simulink library "Chassis_Alpha_org"  (Simulink 10.0)
settings: Solver=ode45  StartTime=0.0  StopTime=10.0  RelTol=1e-3  EnableMultiTasking=on
undefined symbols (not defined in the file): Chassis, lat0, latMean, lon0, Suspension, transMatrix, v_ds, xx_ds, yy_ds, z_accel, z_dist, z_elevTube, z_height
libraries: simulink x4, Chassis_Alpha x2
Description:
  | Copyright 2013-2014 The MathWorks, Inc.
settings Model: Creator=mbrauer  LastModifiedBy=annonymous

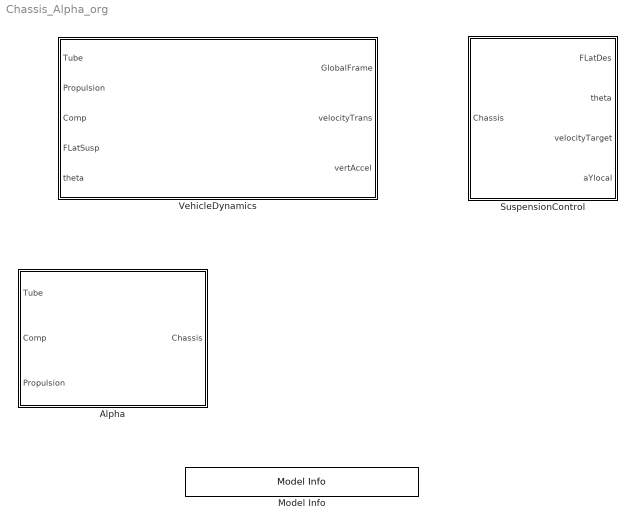
== system Chassis_Alpha_org ==
  Alpha : Subsystem
  Model Info : simulink/Model-Wide Utilities/Model Info  Frame=on  DisplayStringWithTags=%<Description>  HorizontalTextAlignment=Center  LeftAlignmentValue=0.5
  SuspensionControl : Subsystem
  VehicleDynamics : Subsystem

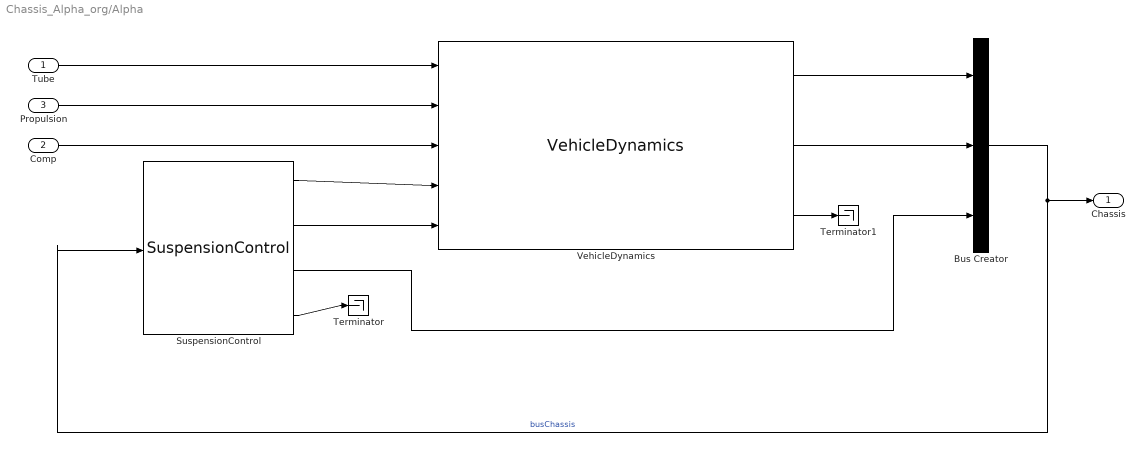
== system Chassis_Alpha_org/Alpha ==
  "Tube " : Inport
  Comp : Inport  Port=2
  Propulsion : Inport  Port=3
  Bus Creator : BusCreator  Inputs=3  NonVirtualBus=on
  SuspensionControl : Chassis_Alpha/SuspensionControl  SystemSampleTime=-1  Latency=0  AutoFrameSizeCalculation=off
  Terminator : Terminator
  Terminator1 : Terminator
  VehicleDynamics : Chassis_Alpha/VehicleDynamics  SystemSampleTime=-1  Latency=0  AutoFrameSizeCalculation=off
  Chassis : Outport
  wires:
  SuspensionControl/4 -> Terminator/1
  Bus Creator/1 -> SuspensionControl/1, Chassis/1  "busChassis"
  Comp/1 -> VehicleDynamics/3
  "Tube "/1 -> VehicleDynamics/1
  VehicleDynamics/1 -> Bus Creator/1
  VehicleDynamics/2 -> Bus Creator/2
  Propulsion/1 -> VehicleDynamics/2
  SuspensionControl/1 -> VehicleDynamics/4
  SuspensionControl/2 -> VehicleDynamics/5
  SuspensionControl/3 -> Bus Creator/3
  VehicleDynamics/3 -> Terminator1/1

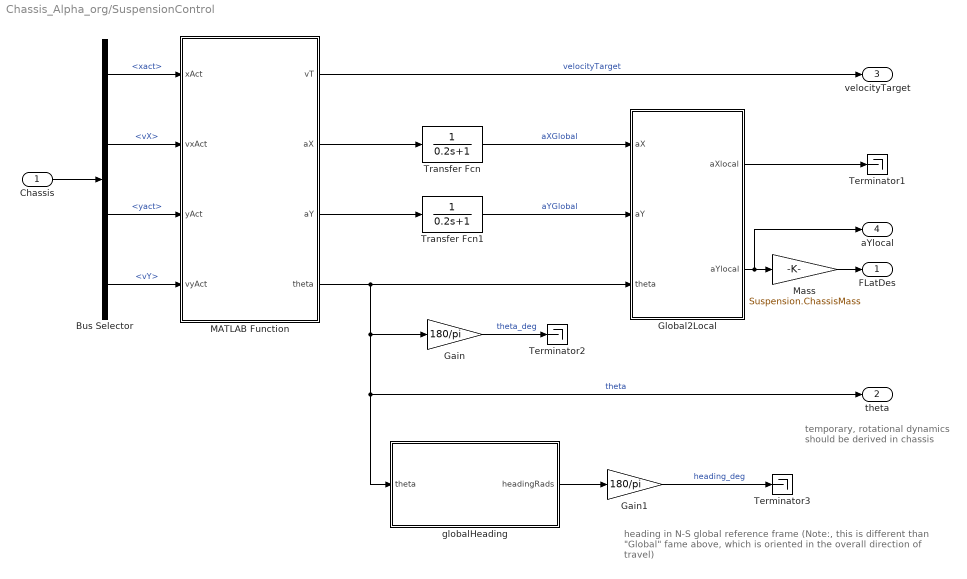
== system Chassis_Alpha_org/SuspensionControl ==
  note: temporary, rotational dynamics
      | should be derived in chassis
  note: heading in N-S global reference frame
      | (Note:, this is different than "Global" fame above, which is oriented
      | in the overall direction of travel)
  Chassis : Inport
  Bus Selector : BusSelector  OutputSignals=GlobalFrame.xact,GlobalFrame.vX,GlobalFrame.yact,GlobalFrame.vY
  Gain : Gain  Gain=180/pi
  Gain1 : Gain  Gain=180/pi
  Global2Local : MATLAB Function  TreatAsAtomicUnit=on
  MATLAB Function : MATLAB Function  TreatAsAtomicUnit=on
  Mass : Gain  Gain=Suspension.ChassisMass
  Terminator1 : Terminator
  Terminator2 : Terminator
  Terminator3 : Terminator
  Transfer Fcn : TransferFcn  Denominator=[0.2 1]
  Transfer Fcn1 : TransferFcn  Denominator=[0.2 1]
  globalHeading : MATLAB Function  TreatAsAtomicUnit=on
  FLatDes : Outport
  theta : Outport  Port=2
  velocityTarget : Outport  Port=3
  aYlocal : Outport  Port=4
  wires:
  Gain1/1 -> Terminator3/1  "heading_deg"
  globalHeading/1(headingRads) -> Gain1/1
  MATLAB Function/2(aX) -> Transfer Fcn/1
  MATLAB Function/3(aY) -> Transfer Fcn1/1
  Transfer Fcn/1 -> Global2Local/1(aX)  "aXGlobal"
  Transfer Fcn1/1 -> Global2Local/2(aY)  "aYGlobal"
  Gain/1 -> Terminator2/1  "theta_deg"
  MATLAB Function/4(theta) -> Gain/1, theta/1, globalHeading/1(theta), Global2Local/3(theta)  "theta"
  Chassis/1 -> Bus Selector/1
  Bus Selector/2 -> MATLAB Function/2(vxAct)  "<vX>"
  Bus Selector/1 -> MATLAB Function/1(xAct)  "<xact>"
  Bus Selector/3 -> MATLAB Function/3(yAct)  "<yact>"
  Bus Selector/4 -> MATLAB Function/4(vyAct)  "<vY>"
  Global2Local/1(aXlocal) -> Terminator1/1
  Global2Local/2(aYlocal) -> Mass/1, aYlocal/1
  Mass/1 -> FLatDes/1
  MATLAB Function/1(vT) -> velocityTarget/1  "velocityTarget"

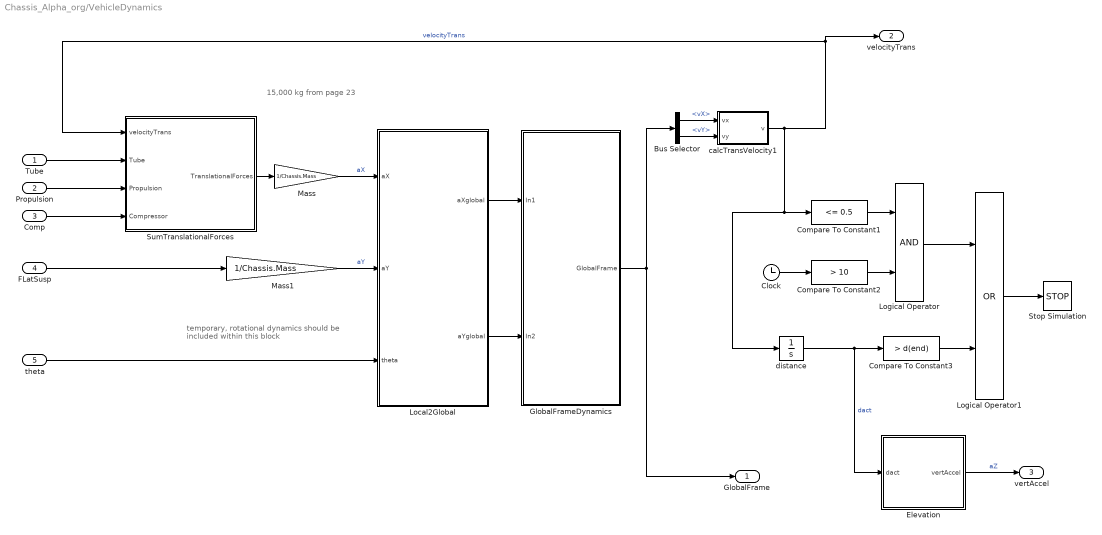
== system Chassis_Alpha_org/VehicleDynamics ==
  note: temporary, rotational dynamics should
      | be included within this block
  note: 15,000 kg from page 23
  "Tube " : Inport
  Propulsion : Inport  Port=2
  Comp : Inport  Port=3
  FLatSusp : Inport  Port=4
  theta : Inport  Port=5
  Bus Selector : BusSelector  OutputSignals=vX,vY
  Clock : Clock
  Compare To Constant1 : simulink/Logic and Bit Operations/Compare To Constant  relop=<=  const=0.5  OutDataTypeStr=boolean
  Compare To Constant2 : simulink/Logic and Bit Operations/Compare To Constant  relop=>  const=10  OutDataTypeStr=boolean  ZeroCross=off
  Compare To Constant3 : simulink/Logic and Bit Operations/Compare To Constant  relop=>  const=d(end)  OutDataTypeStr=boolean  ZeroCross=off
  Elevation : Subsystem
  GlobalFrameDynamics : Subsystem
  Local2Global : MATLAB Function  TreatAsAtomicUnit=on
  Logical Operator : Logic  AllPortsSameDT=off  OutDataTypeStr=boolean
  Logical Operator1 : Logic  Operator=OR  AllPortsSameDT=off  OutDataTypeStr=boolean
  Mass : Gain  Gain=1/Chassis.Mass
  Mass1 : Gain  Gain=1/Chassis.Mass
  Stop Simulation : Stop
  SumTranslationalForces : Subsystem
  calcTransVelocity1 : MATLAB Function  TreatAsAtomicUnit=on
  distance : Integrator
  GlobalFrame : Outport
  velocityTrans : Outport  Port=2
  vertAccel : Outport  Port=3
  wires:
  theta/1 -> Local2Global/3(theta)
  calcTransVelocity1/1(v) -> SumTranslationalForces/1(velocityTrans), velocityTrans/1, Compare To Constant1/1, distance/1  "velocityTrans"
  SumTranslationalForces/1(TranslationalForces) -> Mass/1
  FLatSusp/1 -> Mass1/1
  Mass/1 -> Local2Global/1(aX)  "aX"
  Mass1/1 -> Local2Global/2(aY)  "aY"
  Comp/1 -> SumTranslationalForces/4(Compressor)
  Propulsion/1 -> SumTranslationalForces/3(Propulsion)
  "Tube "/1 -> SumTranslationalForces/2("Tube ")
  distance/1 -> Elevation/1(dact), Compare To Constant3/1  "dact"
  Compare To Constant1/1 -> Logical Operator/1
  Clock/1 -> Compare To Constant2/1
  Compare To Constant2/1 -> Logical Operator/2
  Logical Operator1/1 -> Stop Simulation/1
  Logical Operator/1 -> Logical Operator1/1
  Compare To Constant3/1 -> Logical Operator1/2
  Local2Global/1(aXglobal) -> GlobalFrameDynamics/1(In1)
  Local2Global/2(aYglobal) -> GlobalFrameDynamics/2(In2)
  GlobalFrameDynamics/1(GlobalFrame) -> Bus Selector/1, GlobalFrame/1
  Bus Selector/1 -> calcTransVelocity1/1(vx)  "<vX>"
  Bus Selector/2 -> calcTransVelocity1/2(vy)  "<vY>"
  Elevation/1(vertAccel) -> vertAccel/1  "aZ"

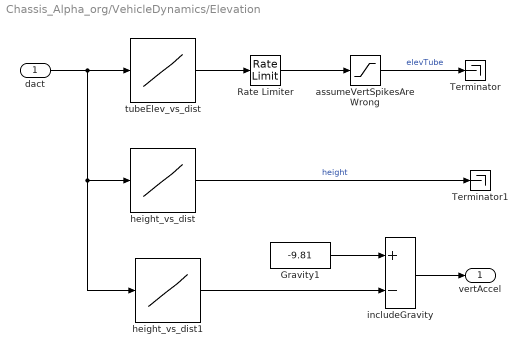
== system Chassis_Alpha_org/VehicleDynamics/Elevation ==
  dact : Inport
  Gravity1 : Constant  Value=-9.81
  Rate Limiter : RateLimiter  RisingSlewLimit=50  FallingSlewLimit=-50  SampleTimeMode=inherited
  Terminator : Terminator
  Terminator1 : Terminator
  assumeVertSpikesAreWrong : Saturate  UpperLimit=5  LowerLimit=-5
  height_vs_dist : Lookup_n-D  NumberOfTableDimensions=1  BreakpointsForDimension1=z_dist  BeginIndexSearchUsingPreviousIndexResult=on  Table=z_height  ExtrapMethod=Clip  InternalRulePriority=Speed  RndMeth=Simplest  InputSameDT=on
  height_vs_dist1 : Lookup_n-D  NumberOfTableDimensions=1  BreakpointsForDimension1=z_dist  BeginIndexSearchUsingPreviousIndexResult=on  Table=z_accel  ExtrapMethod=Clip  InternalRulePriority=Speed  RndMeth=Simplest  InputSameDT=on
  includeGravity : Sum  Inputs=+-
  tubeElev_vs_dist : Lookup_n-D  NumberOfTableDimensions=1  BreakpointsForDimension1=z_dist  BeginIndexSearchUsingPreviousIndexResult=on  Table=z_elevTube  InternalRulePriority=Speed  RndMeth=Simplest  InputSameDT=on
  vertAccel : Outport
  wires:
  dact/1 -> tubeElev_vs_dist/1, height_vs_dist1/1, height_vs_dist/1
  assumeVertSpikesAreWrong/1 -> Terminator/1  "elevTube"
  height_vs_dist/1 -> Terminator1/1  "height"
  Gravity1/1 -> includeGravity/1
  includeGravity/1 -> vertAccel/1
  tubeElev_vs_dist/1 -> Rate Limiter/1
  Rate Limiter/1 -> assumeVertSpikesAreWrong/1
  height_vs_dist1/1 -> includeGravity/2

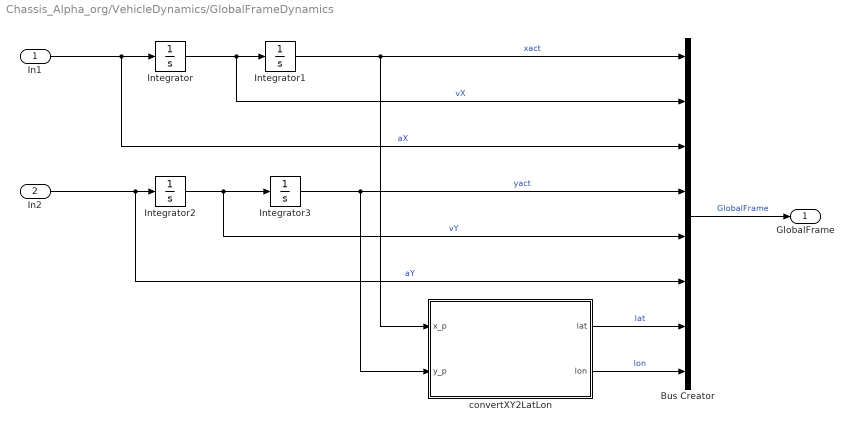
== system Chassis_Alpha_org/VehicleDynamics/GlobalFrameDynamics ==
  In1 : Inport
  In2 : Inport  Port=2
  Bus Creator : BusCreator  Inputs=8
  Integrator{,1..3} (4 alike) : Integrator
  convertXY2LatLon : MATLAB Function  TreatAsAtomicUnit=on
  GlobalFrame : Outport
  wires:
  Integrator/1 -> Bus Creator/2, Integrator1/1  "vX"
  In2/1 -> Bus Creator/6, Integrator2/1  "aY"
  Integrator1/1 -> convertXY2LatLon/1(x_p), Bus Creator/1  "xact"
  Integrator3/1 -> convertXY2LatLon/2(y_p), Bus Creator/4  "yact"
  In1/1 -> Bus Creator/3, Integrator/1  "aX"
  Integrator2/1 -> Bus Creator/5, Integrator3/1  "vY"
  Bus Creator/1 -> GlobalFrame/1  "GlobalFrame"
  convertXY2LatLon/1(lat) -> Bus Creator/7  "lat"
  convertXY2LatLon/2(lon) -> Bus Creator/8  "lon"

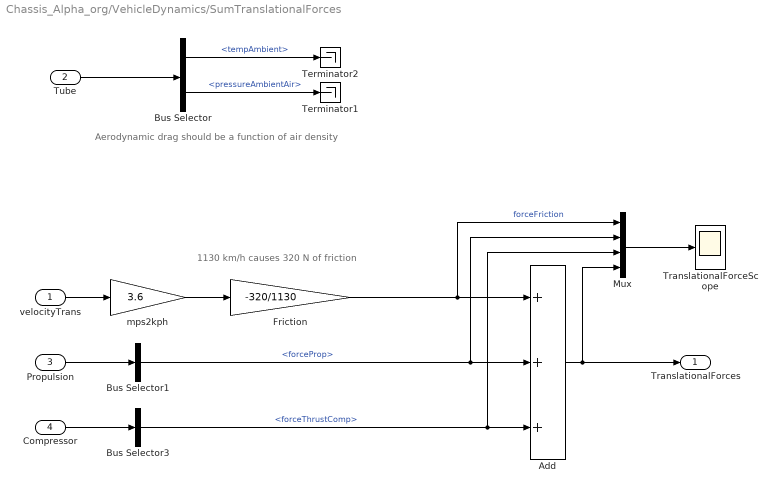
== system Chassis_Alpha_org/VehicleDynamics/SumTranslationalForces ==
  note: Aerodynamic drag should be a function of air density
  note: 1130 km/h causes 320 N of friction
  velocityTrans : Inport
  "Tube " : Inport  Port=2
  Propulsion : Inport  Port=3
  Compressor : Inport  Port=4
  Add : Sum  Inputs=+++
  Bus Selector : BusSelector  OutputSignals=tempAmbient,pressureAmbientAir
  Bus Selector1 : BusSelector  OutputSignals=forceProp
  Bus Selector3 : BusSelector  OutputSignals=forceThrustComp
  Friction : Gain  Gain=-320/1130
  Mux : Mux
  Terminator1 : Terminator
  Terminator2 : Terminator
  TranslationalForceScope : Scope
  mps2kph : Gain  Gain=3.6
  TranslationalForces : Outport
  wires:
  velocityTrans/1 -> mps2kph/1
  "Tube "/1 -> Bus Selector/1
  Bus Selector/1 -> Terminator2/1  "<tempAmbient>"
  Bus Selector/2 -> Terminator1/1  "<pressureAmbientAir>"
  mps2kph/1 -> Friction/1
  Propulsion/1 -> Bus Selector1/1
  Compressor/1 -> Bus Selector3/1
  Bus Selector1/1 -> Mux/2, Add/2  "<forceProp>"
  Bus Selector3/1 -> Mux/3, Add/3  "<forceThrustComp>"
  Mux/1 -> TranslationalForceScope/1
  Add/1 -> TranslationalForces/1, Mux/4
  Friction/1 -> Mux/1, Add/1  "forceFriction"

== matlab function VehicleDynamics/GlobalFrameDynamics/convertXY2LatLon ==
  data: x_p input double; lat output double; y_p input double; transMatrix parameter double; lat0 parameter double; lon0 parameter double; lon output double; latMean parameter double
function [lat, lon ] = convertXY2LatLon(x_p,y_p,transMatrix,lat0,lon0, latMean)
%reorientXY2LatLon  re-orient a single cartesian data point to latitude 
% and longitude in degrees. The translation matrix, which was used 
% to do the opposite conversion, is required.
%
%   Copyright 2013 - 2014 The MathWorks, Inc

%% Re-orient based on original transMatrix
x_y_p   = [x_p';y_p'];
x_y     = transMatrix\x_y_p;
x_p     = x_y(1,:)';
y_p     = x_y(2,:)';

%% Convert cartesian coordinates to latitude and longitude 
LatLon2Met.Lat      = [30      35      40       45      50];
LatLon2Met.Lat2Met  = [110852  110940  111035   111132  111229];
LatLon2Met.Lon2Met  = [96486   91288   85394    78847   71696];

% Determine conversion at everage latitude
lat2met = interp1(LatLon2Met.Lat,LatLon2Met.Lat2Met,latMean);
lon2met = interp1(LatLon2Met.Lat,LatLon2Met.Lon2Met,latMean);

lon     = x_p/lon2met+lon0;
lat     = y_p/lat2met+lat0;

== matlab function SuspensionControl/Global2Local ==
  data: aX input double; aY input double; theta input double; aXlocal output double; aYlocal output double
function [aXlocal, aYlocal]  = global2Local(aX,aY, theta)

transMatrix = [cos(theta) sin(theta);-sin(theta) cos(theta)];
aLocal      = transMatrix*[aX;aY];
aXlocal     = aLocal(1);
aYlocal     = aLocal(2);

== matlab function VehicleDynamics/Local2Global ==
  data: aX input double; aY input double; theta input double; aXglobal output double; aYglobal output double
function [aXglobal, aYglobal]  = Local2Global(aX,aY, theta)

transMatrix     = [cos(theta) sin(theta);-sin(theta) cos(theta)];
transMatrixInv  = inv(transMatrix);
aGlobal         = transMatrixInv*[aX;aY];
aXglobal        = aGlobal(1);
aYglobal        = aGlobal(2);

== matlab function SuspensionControl/MATLAB Function ==
  data: vT output double; xAct input double; vxAct input double; aX output double; yAct input double; vyAct input double; xx_ds parameter double; yy_ds parameter double; v_ds parameter double; aY output double; theta output double
function [vT, aX, aY, theta] = findIdealTraj(xAct, vxAct, yAct, vyAct, xx_ds, yy_ds, v_ds)
% determines the desired acceleration in x and y direction given an actual
% position (xAct, yAct) and velocity (vxAct, vyAct) with parameters of 
% ideal trajectory (xx_ds, yy_ds) and velocity (v_ds) profiles

%% Find index of next closest point in trajectory (not necessarily the closest)
% Find closest point
distToRouteX        = xx_ds - ones(size(xx_ds))*xAct;
distToRouteY        = yy_ds - ones(size(xx_ds))*yAct;
distToRoute         = sqrt(distToRouteX.^2+distToRouteY.^2);
[distToPoint, idxA] = min(distToRoute);   % idxA corresponds to closest point

% find next nearest point that isn't too close       
if idxA == 1
    idx = 2;                    % just getting started
elseif idxA == length(xx_ds)
    idx = idxA;        % last point
elseif distToPoint < 60; % if very close to the point, use the next point
    idx = idxA + 1;
else                % either the closest point or the point after it is next
    distToRoute_nearest = [distToRoute(idxA-1) distToRoute(idxA+1)]; 
    [~, idx_rel] = min(distToRoute_nearest);
    idx = idxA +idx_rel - 1; % idx_rel = 1, idx is idxA (next point is nearest)
                         % idx_rel = 2, idx is idxA + 1 (next point is after nearest)
end                   

if idx>length(xx_ds)
    error('index exceeds length of xx_ds')
end

%% Determine desired acceleration
% give default values for output values to make MATLAB happy
aX      = 0;
aY      = 0;
tau1    = [1;0];        
vT      = 0;

% Move target point out until necessary acelaration is below a limit
flagExtendView  = true;
maxAccel        = 15;  % m/s2

while flagExtendView

% Distance vector to next point
deltaX1 = xx_ds(idx) - xAct;
deltaY1 = yy_ds(idx) - yAct;
dist    = sqrt(deltaX1^2+deltaY1^2);
tau1    = [deltaX1;deltaY1];
tauNorm1= tau1/norm(tau1);

% Distance vector to point after next (to determine tanjential velocity at
% next point)
if idx == length(xx_ds)    % last point so just extend direction
    tauNorm2 = tauNorm1;    
else
    deltaX2 = xx_ds(idx+1) - xx_ds(idx);
    deltaY2 = yy_ds(idx+1) - yy_ds(idx);
    tau2    = [deltaX2;deltaY2];
    tauNorm2= tau2/norm(tau2);
end

% Velocity vector at next point
if and(any(isnan(tauNorm1)),any(isnan(tauNorm2)))
    vTemp = [1 1];  % this shouldn't happen
%     warning('duplicate route points found at index = %d',idx)
elseif any(isnan(tauNorm1))
    vTemp = tauNorm2;
elseif any(isnan(tauNorm2))
    vTemp = tauNorm1;
else
    vTemp   = mean([tauNorm1,tauNorm2],2); % take mean of direction vectors
end
vTemp   = vTemp/norm(vTemp);           % re-normalize (magnitude of 1)
vVec    = v_ds(idx)*vTemp;             % mutiply by velocity magnitude
vT      = sqrt(vVec(1)^2+vVec(2)^2);
      
% Acceleration      
vAct    = sqrt(vxAct^2+vyAct^2);       % current velocity magnitude
time    = 2*dist/(vAct+v_ds(idx));     % time to reach next point
aX      = (vVec(1) - vxAct)/time;   
aY      = (vVec(2) - vyAct)/time; 

if idx == length(xx_ds)  % last point, need to accept acceleration target
    flagExtendView = false;
elseif sqrt(aX^2+aY^2)>maxAccel;
    idx = idx + 1; 
else
    flagExtendView = false;
end

end

%% Determine local orientation of vehicle
if and(vyAct==0,vxAct==0)
    theta = atan2(tau1(2),tau1(1));
else
    theta = atan2(vyAct,vxAct);
end

== matlab function VehicleDynamics/calcTransVelocity1 ==
  data: vx input double; v output double; vy input double
function v = fcn(vx,vy)
v = (vx^2+vy^2)^0.5;

== matlab function SuspensionControl/globalHeading ==
  data: theta input double; transMatrix parameter double; headingRads output double
function headingRads   = globalHeading(theta, transMatrix)

forwardLocal        = [1;0];
transMatrixLocal    = [cos(theta) sin(theta);-sin(theta) cos(theta)];
headingVector       = inv(transMatrix)*inv(transMatrixLocal)*forwardLocal;
headingRads         = atan2(headingVector(2),headingVector(1));
            % 0 deg is facing E. 
            % 90 is N
            % -90 is S
            % 180 or -180 is W
